simulink model "petosaalis"  (R2020b)
settings: Solver=VariableStepAuto  StartTime=0.0  StopTime=10.0  MaxStep=0.01  RelTol=1e-3
settings Model: Creator=kiisk  LastModifiedBy=kiisk

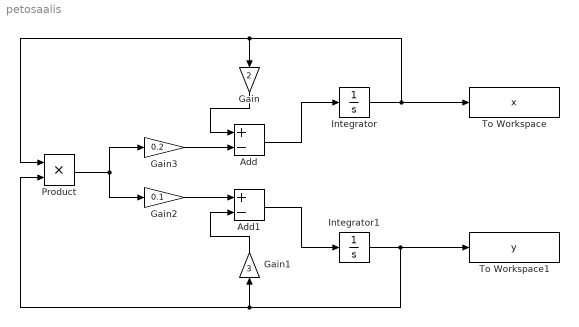
== system petosaalis ==
  Add : Sum  Inputs=+-
  Add1 : Sum  Inputs=+-
  Gain : Gain  Gain=2
  Gain1 : Gain  Gain=3
  Gain2 : Gain  Gain=0.1
  Gain3 : Gain  Gain=0.2
  Integrator : Integrator  InitialCondition=5
  Integrator1 : Integrator  InitialCondition=2
  Product : Product
  To Workspace : ToWorkspace  VariableName=x  SampleTime=-1
  To Workspace1 : ToWorkspace  VariableName=y  SampleTime=-1
  wires:
  Integrator/1 -> To Workspace/1, Gain/1, Product/1
  Integrator1/1 -> To Workspace1/1, Gain1/1, Product/2
  Gain/1 -> Add/1
  Gain1/1 -> Add1/2
  Product/1 -> Gain2/1, Gain3/1
  Gain3/1 -> Add/2
  Gain2/1 -> Add1/1
  Add/1 -> Integrator/1
  Add1/1 -> Integrator1/1
